simulink model "pwm_delayed_pred_noised_controlled_system"  (R2017a)
settings: Solver=VariableStepAuto  StartTime=0.0  StopTime=t_f  RelTol=1e-3
values from neighbouring files (symbols this model uses):
  C_ = C    [load_delay.m]
  Ctilde = [Ctilde, zeros(n_Ctilde, s_nds_i)]    [load_delay.m]    (also in load_pwm_delayed_controller.m = Ctilde(1, 1:2); load_pwm_delayed_pred_controller.m = Ctilde(1, 1:2); load_pwm_pred_controller.m = Ctilde(1:2))
  mean_val = 0    [load_pwm_delayed_pred_noised_controller.m]
  step_ref = torque_ref    [sim_controlled_system.m]
  var_val = 0.5    [load_pwm_delayed_pred_noised_controller.m]
  x0 = [0; 0]    [sim_controlled_system.m]
undefined symbols (not defined in the file or in its folder): A, B, Tpwm_val, Ts_val, Vcc_val
settings Model: Creator=brunolnetto  LastModifiedBy=brunolnetto
settings SolverCC: AlgebraicLoopSolver=LineSearch

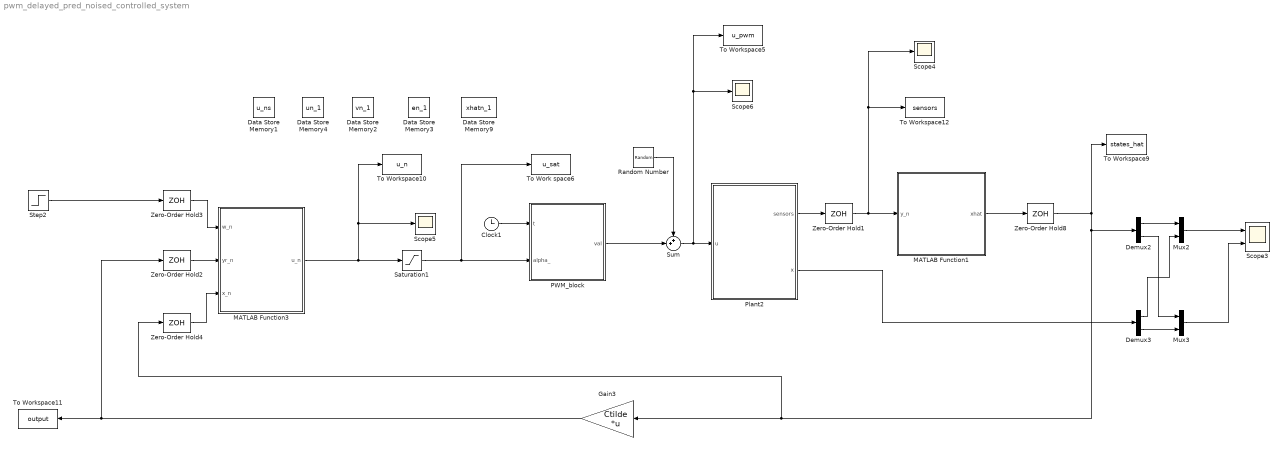
== system pwm_delayed_pred_noised_controlled_system ==
  Clock1 : Clock
  Data Store Memory1 : DataStoreMemory  DataStoreName=u_ns  ReadBeforeWriteMsg=warning  WriteAfterWriteMsg=warning  WriteAfterReadMsg=warning  InitialValue=u_ns0  ShowAdditionalParam=off  OutDataTypeStr=double
  Data Store Memory2 : DataStoreMemory  DataStoreName=vn_1  ReadBeforeWriteMsg=warning  WriteAfterWriteMsg=warning  WriteAfterReadMsg=warning  ShowAdditionalParam=off  OutDataTypeStr=double
  Data Store Memory3 : DataStoreMemory  DataStoreName=en_1  ReadBeforeWriteMsg=warning  WriteAfterWriteMsg=warning  WriteAfterReadMsg=warning  InitialValue=e0  ShowAdditionalParam=off  OutDataTypeStr=double
  Data Store Memory4 : DataStoreMemory  DataStoreName=un_1  ReadBeforeWriteMsg=warning  WriteAfterWriteMsg=warning  WriteAfterReadMsg=warning  ShowAdditionalParam=off  OutDataTypeStr=double
  Data Store Memory9 : DataStoreMemory  DataStoreName=xhatn_1  ReadBeforeWriteMsg=warning  WriteAfterWriteMsg=warning  WriteAfterReadMsg=warning  InitialValue=xhat0  ShowAdditionalParam=off  OutDataTypeStr=double
  Demux2 : Demux  Outputs=2
  Demux3 : Demux  Outputs=2
  Gain3 : Gain  Gain=Ctilde  Multiplication=Matrix(K*u) (u vector)
  MATLAB Function1 : MATLAB Function  TreatAsAtomicUnit=on
  MATLAB Function3 : MATLAB Function  TreatAsAtomicUnit=on
  Mux2 : Mux  Inputs=2
  Mux3 : Mux  Inputs=2
  PWM_block : MATLAB Function  TreatAsAtomicUnit=on
  Plant2 : Subsystem
  Random Number : RandomNumber  Mean=mean_val  Variance=var_val
  Saturation1 : Saturate  UpperLimit=1  LowerLimit=-1
  Scope3 : Scope  NumInputPorts=2
  Scope4 : Scope
  Scope5 : Scope
  Scope6 : Scope
  Step2 : Step  Time=0  After=step_ref  SampleTime=Ts_val
  Sum : Sum  Inputs=++|
  To Work space6 : ToWorkspace  VariableName=u_sat  SaveFormat=Structure With Time  SampleTime=-1
  To Workspace10 : ToWorkspace  VariableName=u_n  SaveFormat=Structure With Time  SampleTime=-1
  To Workspace11 : ToWorkspace  VariableName=output  SaveFormat=Structure With Time  SampleTime=-1
  To Workspace12 : ToWorkspace  VariableName=sensors  SaveFormat=Structure With Time  SampleTime=-1
  To Workspace5 : ToWorkspace  VariableName=u_pwm  SaveFormat=Structure With Time  SampleTime=-1
  To Workspace9 : ToWorkspace  VariableName=states_hat  SaveFormat=Structure With Time  SampleTime=-1
  Zero-Order Hold{1..4,8} (5 alike) : ZeroOrderHold  SampleTime=Ts_val
  wires:
  Plant2/1(sensors) -> Zero-Order Hold1/1
  Zero-Order Hold2/1 -> MATLAB Function3/2(yr_n)
  PWM_block/1(val) -> Sum/2
  Clock1/1 -> PWM_block/1(t)
  Demux3/1 -> Mux2/2
  Zero-Order Hold3/1 -> MATLAB Function3/1(w_n)
  Step2/1 -> Zero-Order Hold3/1
  Saturation1/1 -> To Work space6/1, PWM_block/2(alpha_)
  Gain3/1 -> Zero-Order Hold2/1, To Workspace11/1
  Zero-Order Hold8/1 -> Demux2/1, Zero-Order Hold4/1, Gain3/1, To Workspace9/1
  Demux2/1 -> Mux2/1
  Zero-Order Hold1/1 -> MATLAB Function1/1(y_n), Scope4/1, To Workspace12/1
  Mux2/1 -> Scope3/1
  Zero-Order Hold4/1 -> MATLAB Function3/3(x_n)
  MATLAB Function1/1(xhat) -> Zero-Order Hold8/1
  Demux2/2 -> Mux3/1
  Mux3/1 -> Scope3/2
  Plant2/2(x) -> Demux3/1
  Demux3/2 -> Mux3/2
  MATLAB Function3/1(u_n) -> Scope5/1, To Workspace10/1, Saturation1/1
  Random Number/1 -> Sum/1
  Sum/1 -> To Workspace5/1, Scope6/1, Plant2/1(u)

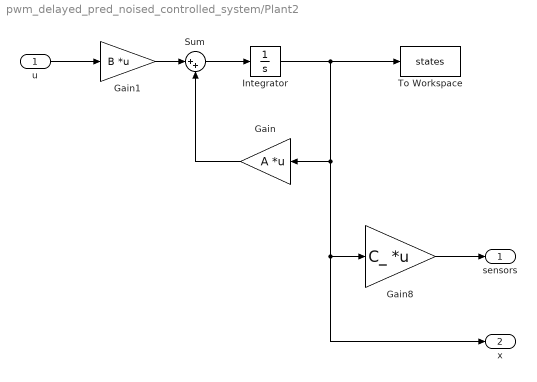
== system pwm_delayed_pred_noised_controlled_system/Plant2 ==
  u : Inport
  Gain : Gain  Gain=A  Multiplication=Matrix(K*u) (u vector)
  Gain1 : Gain  Gain=B  Multiplication=Matrix(K*u) (u vector)
  Gain8 : Gain  Gain=C_  Multiplication=Matrix(K*u) (u vector)
  Integrator : Integrator  InitialCondition=x0
  Sum : Sum  Inputs=|++
  To Workspace : ToWorkspace  VariableName=states  SaveFormat=Structure With Time  SampleTime=-1
  sensors : Outport
  x : Outport  Port=2
  wires:
  Gain8/1 -> sensors/1
  Gain1/1 -> Sum/1
  u/1 -> Gain1/1
  Gain/1 -> Sum/2
  Sum/1 -> Integrator/1
  Integrator/1 -> To Workspace/1, x/1, Gain8/1, Gain/1

== matlab function pwm_delayed_pred_noised_controlled_system/MATLAB Function1 ==
  data: y_n input; xhat output; un_1 data_store_memory; xhatn_1 data_store_memory; params parameter
function xhat = observador (y_n, params)
    global un_1;
    global xhatn_1;
    
%     x_bar = params.Phi*xhatn_1 + params.Gamma*un_1;
%     xhat = x_bar + params.L*(y - params.C*xhatn_1);
    
    Phi = params.Phi;
    Gamma = params.Gamma;
    L = params.L;
    C = params.C;

    xhat = Phi*xhatn_1 + Gamma*un_1 + L*(y_n - C*xhatn_1);

    xhatn_1 = xhat;
end

== matlab function pwm_delayed_pred_noised_controlled_system/MATLAB Function3 ==
  data: w_n input; yr_n input; x_n input; u_n output; vn_1 data_store_memory; params parameter; en_1 data_store_memory; un_1 data_store_memory; u_ns data_store_memory
function u_n = controller(w_n, yr_n, x_n, params)
    global vn_1;
    global en_1;
    global un_1;
    global u_ns;
    
    x_n = [x_n; u_ns];    
    v_n = vn_1 + en_1;
    
    u_i = params.Ki*v_n;
    u_p = - params.Kp*x_n;
    
    u_n = u_i + u_p;
    
    vn_1 = v_n;
    en_1 = w_n - yr_n;
    un_1 = u_n;
    u_ns = [u_n; u_ns(2:end)];
end

== matlab function pwm_delayed_pred_noised_controlled_system/PWM_block ==
  data: t input; alpha_ input; val output; Vcc_val parameter; Tpwm_val parameter
function val = pwm_signal(t, alpha_, Vcc_val, Tpwm_val)
    % Static variable
    persistent t0;
    
    if(isempty(t0))
        t0 = 0;
    end
        
    % PWM generation
    if(t == 0)
        t0 = 0;
    end
    
    if(t - t0 > Tpwm_val)
        t0 = t;
    end
    
    % Inner time interval
    t_i = t - t0;
    
    abs_alpha = abs(alpha_);
    sign_alpha = sign(alpha_);
    
    if(t_i <= abs_alpha*Tpwm_val)
        val = sign_alpha*Vcc_val;
    else
        val = 0;
    end
end
